simulink model "analog__mod"  (R2023a)
settings: Solver=VariableStepAuto  StartTime=0.0  StopTime=16  MaxStep=0.0001  RelTol=1e-3
settings Model: Creator=tanov  LastModifiedBy=tanov

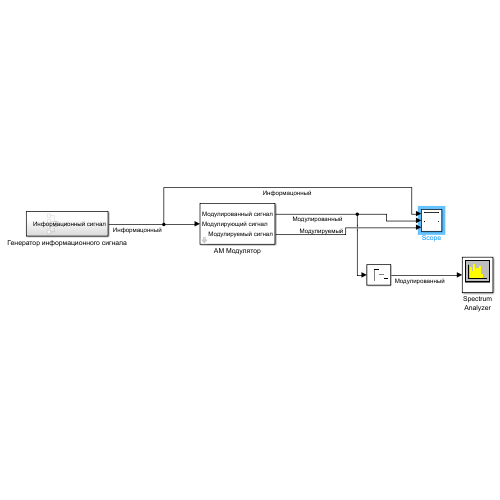
[thumbnail: Simulink's stored preview of the top-level diagram]
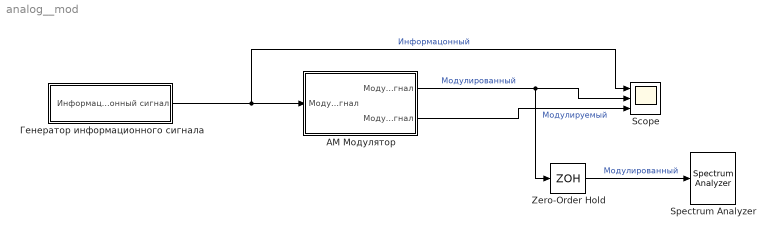
== system analog__mod ==
  AM Модулятор : Subsystem  mask{f_c=300, m=1.5}
      mask prompts: f_c "Частота несущей"; m "Порядок модуляции"
  Scope : Scope  NumInputPorts=3
  Spectrum Analyzer : SpectrumAnalyzer  WindowPosition=[1.000000,49.000000,1600.000000,930.000000,]  ScopeFrameLocation=window  Span=1000  StartFrequency=-500  StopFrequency=500  YLimits=[-78.2961378,33.85431457]  ColorLimits=[-20 80]  DefaultConfigurationName=spbscopes.SpectrumAnalyzerBlockCfg  IsFrequencyInputMode=0  FrequencyVectorPort=0  FrequencyVectorFromPort=0  FrequencyInputRBWPort=0  FrequencyInputRBWFromPort=0
  Zero-Order Hold : ZeroOrderHold  SampleTime=1e-3
  Генератор информационного сигнала : Subsystem
  wires:
  Генератор информационного сигнала/1(Информационный сигнал) -> Scope/1, AM Модулятор/1(Модулирующий сигнал)  "Информацонный"
  AM Модулятор/2(Модулируемый сигнал) -> Scope/3  "Модулируемый"
  AM Модулятор/1(Модулированный сигнал) -> Zero-Order Hold/1, Scope/2  "Модулированный"
  Zero-Order Hold/1 -> Spectrum Analyzer/1  "Модулированный"

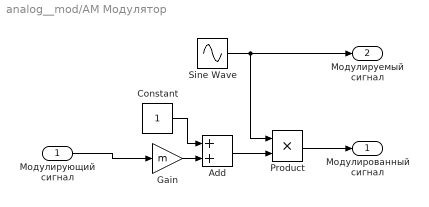
== system analog__mod/AM Модулятор ==
  Модулирующий сигнал : Inport
  Add : Sum
  Constant : Constant
  Gain : Gain  Gain=m
  Product : Product
  Sine Wave : Sin  Frequency=2*pi*f_c  Phase=pi/2  SampleTime=0
  Модулированный сигнал : Outport
  Модулируемый сигнал : Outport  Port=2
  wires:
  Sine Wave/1 -> Product/1, Модулируемый сигнал/1
  Модулирующий сигнал/1 -> Gain/1
  Gain/1 -> Add/2
  Constant/1 -> Add/1
  Add/1 -> Product/2
  Product/1 -> Модулированный сигнал/1

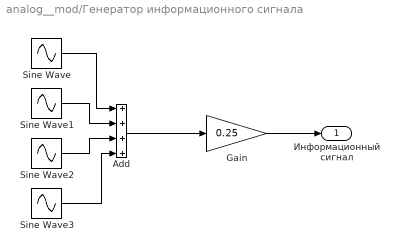
== system analog__mod/Генератор информационного сигнала ==
  Add : Sum  Inputs=++++
  Gain : Gain  Gain=0.25
  Sine Wave : Sin  Frequency=2*pi*40  SampleTime=0
  Sine Wave1 : Sin  Frequency=2*pi*60  SampleTime=0
  Sine Wave2 : Sin  Frequency=2*pi*80  SampleTime=0
  Sine Wave3 : Sin  Frequency=2*pi*100  SampleTime=0
  Информационный сигнал : Outport
  wires:
  Sine Wave/1 -> Add/1
  Sine Wave3/1 -> Add/4
  Sine Wave1/1 -> Add/2
  Sine Wave2/1 -> Add/3
  Add/1 -> Gain/1
  Gain/1 -> Информационный сигнал/1
